simulink model "Simulation_Model1"  (R2020a)
settings: Solver=FixedStepAuto  StartTime=0.0  StopTime=6  FixedStep=.01  RelTol=1e-3
values from neighbouring files (symbols this model uses):
  Mot = F15_Motor    [Simulation_Init.m]
  Veh = Vehicle    [Simulation_Init.m]
libraries: simulink x4, Drag_ul x1, Gravity_ul x1, CgCp_ul x1, NormalForce_ul x1, ThrustCurve_ul x1, Environment_cl x1, Scope_ul x1
settings Model: Creator=bunce  LastModifiedBy=bunce
settings DataIOCC: ReturnWorkspaceOutputs=off
settings SFSimCC: CustomCodeUndefinedFunction=UseInterfaceOnly

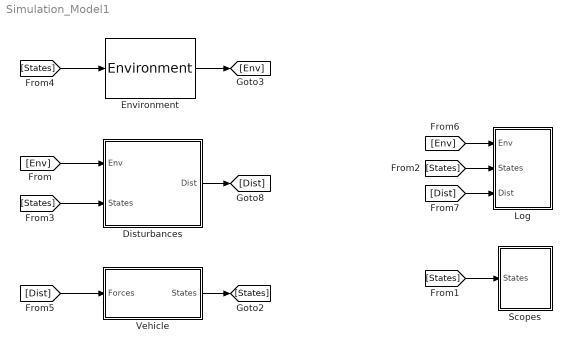
== system Simulation_Model1 ==
  Disturbances : Subsystem
      mask Display:
      | patch([0 1 1 0], [0 0 1 1],[1 .85 1])
      | 
      | port_label('input',1,'Env','texmode','on')
      | 
      | port_label('input',2,'States','texmode','on')
      | 
      | port_label('output',1,'Dist','texmode','on')
  Environment : Environment_cl/Environment  SystemSampleTime=-1  Latency=0  AutoFrameSizeCalculation=off
  Log : Subsystem
      mask Display:
      | patch([0 1 1 0], [0 0 1 1],[1 .85 1])
      | 
      | port_label('input',1,'Env','texmode','on')
      | 
      | port_label('input',2,'States','texmode','on')
      | 
      | port_label('input',3,'Dist','texmode','on')
  Scopes : Subsystem
      mask Display:
      | patch([0 1 1 0], [0 0 1 1],[1 .85 1])
      | 
      | port_label('input',1,'States','texmode','on')
  Vehicle : Subsystem
  wires:
  [Dist] -> Vehicle/1("Forces ")
  Vehicle/1("States ") -> [States]
  [Env] -> Disturbances/1("Env ")
  [States] -> Disturbances/2("States ")
  Disturbances/1(Dist) -> [Dist]
  Environment/1 -> [Env]
  [States] -> Environment/1
  [Dist] -> Log/3(Dist)
  [States] -> Log/2(States)
  [Env] -> Log/1(Env)
  [States] -> Scopes/1(States)

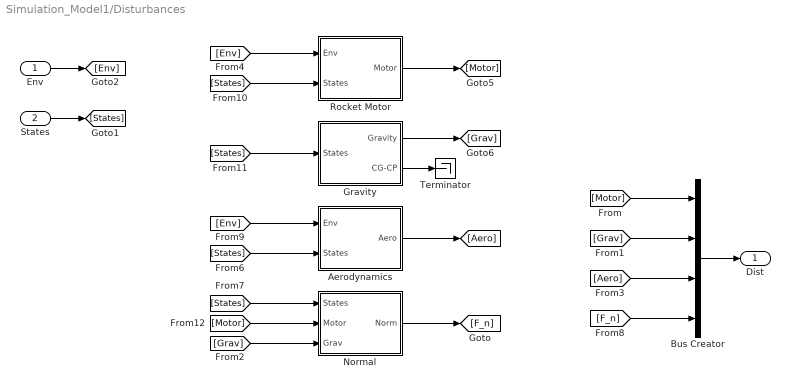
== system Simulation_Model1/Disturbances ==
  "Env " : Inport
  "States " : Inport  Port=2
  Aerodynamics : Subsystem
      mask Display:
      | patch([0 1 1 0], [0 0 1 1],[1 .85 1])
      | 
      | port_label('input',1,'Env','texmode','on')
      | 
      | port_label('input',2,'States', 'texmode','on')
      | 
      | port_label('output',1,'Aero','texmode','on')
  Bus Creator : BusCreator  Inputs=4
  Gravity : Subsystem
      mask Display:
      | patch([0 1 1 0], [0 0 1 1],[1 .85 1])
      | 
      | port_label('input',1,'States','texmode','on')
      | 
      | 
      | port_label('output',1,'Grav','texmode','on')
      | 
      | port_label('output',2,'CG-CP','texmode','on')
  Normal : Subsystem
      mask Display:
      | patch([0 1 1 0], [0 0 1 1],[1 .85 1])
      | 
      | port_label('input',1,'States','texmode','on')
      | 
      | port_label('input',2,'Motor', 'texmode','on')
      | 
      | port_label('input',3,'Grav', 'texmode','on')
      | 
      | port_label('output',1,'F_n','texmode','on')
  Rocket Motor : Subsystem
      mask Display:
      | patch([0 1 1 0], [0 0 1 1],[1 .85 1])
      | 
      | port_label('input',1,'Env','texmode','on')
      | 
      | port_label('input',2,'States', 'texmode','on')
      | 
      | port_label('output',1,'Motor','texmode','on')
  Terminator : Terminator
  Dist : Outport  VectorParamsAs1DForOutWhenUnconnected=off
  wires:
  "States "/1 -> [States]
  [Motor] -> Bus Creator/1
  [Grav] -> Bus Creator/2
  [Aero] -> Bus Creator/3
  [F_n] -> Bus Creator/4
  Bus Creator/1 -> Dist/1
  "Env "/1 -> [Env]
  [States] -> Aerodynamics/2(States)
  [Env] -> Aerodynamics/1(Env)
  Aerodynamics/1(Aero) -> [Aero]
  [Env] -> Rocket Motor/1(Env)
  Rocket Motor/1(Motor) -> [Motor]
  [States] -> Rocket Motor/2(States)
  Gravity/1(Gravity) -> [Grav]
  [States] -> Gravity/1(States)
  [States] -> Normal/1(States)
  [Motor] -> Normal/2(Motor)
  [Grav] -> Normal/3(Grav)
  Normal/1(Norm) -> [F_n]
  Gravity/2(CG-CP) -> Terminator/1

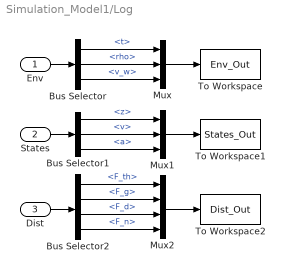
== system Simulation_Model1/Log ==
  Env : Inport
  States : Inport  Port=2
  Dist : Inport  Port=3
  Bus Selector : BusSelector  OutputSignals=t,rho,v_w
  Bus Selector1 : BusSelector  OutputSignals=z,v,a
  Bus Selector2 : BusSelector  OutputSignals=Motor.F_th,Gravity.F_g,Aero.F_d,Norm.F_n
  Mux : Mux  Inputs=3
  Mux1 : Mux  Inputs=3
  Mux2 : Mux
  To Workspace : ToWorkspace  VariableName=Env_Out  SaveFormat=Structure With Time  SampleTime=-1
  To Workspace1 : ToWorkspace  VariableName=States_Out  SaveFormat=Structure With Time  SampleTime=-1
  To Workspace2 : ToWorkspace  VariableName=Dist_Out  SaveFormat=Structure With Time  SampleTime=-1
  wires:
  Env/1 -> Bus Selector/1
  States/1 -> Bus Selector1/1
  Dist/1 -> Bus Selector2/1
  Bus Selector1/3 -> Mux1/3  "<a>"
  Bus Selector1/2 -> Mux1/2  "<v>"
  Bus Selector2/2 -> Mux2/2  "<F_g>"
  Bus Selector2/3 -> Mux2/3  "<F_d>"
  Bus Selector2/4 -> Mux2/4  "<F_n>"
  Bus Selector2/1 -> Mux2/1  "<F_th>"
  Bus Selector1/1 -> Mux1/1  "<z>"
  Bus Selector/1 -> Mux/1  "<t>"
  Bus Selector/2 -> Mux/2  "<rho>"
  Bus Selector/3 -> Mux/3  "<v_w>"
  Mux/1 -> To Workspace/1
  Mux1/1 -> To Workspace1/1
  Mux2/1 -> To Workspace2/1

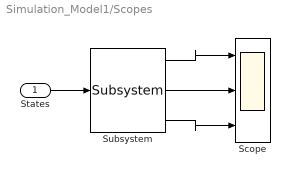
== system Simulation_Model1/Scopes ==
  States : Inport
  Scope : Scope  NumInputPorts=3
  Subsystem : Scope_ul/Subsystem  SystemSampleTime=-1  Latency=0  AutoFrameSizeCalculation=off
      mask Display:
      | patch([0 1 1 0], [0 0 1 1],[.8 1 1])
      | 
      | port_label('input',1,'States','texmode','on')
      | 
      | port_label('output',1,'z [m]','texmode','on')
      | 
      | port_label('output',2,'v [m/s]','texmode','on')
      | 
      | port_label('output',3,'a [m/s^2]','texmode','on')
  wires:
  States/1 -> Subsystem/1
  Subsystem/1 -> Scope/1
  Subsystem/2 -> Scope/2
  Subsystem/3 -> Scope/3

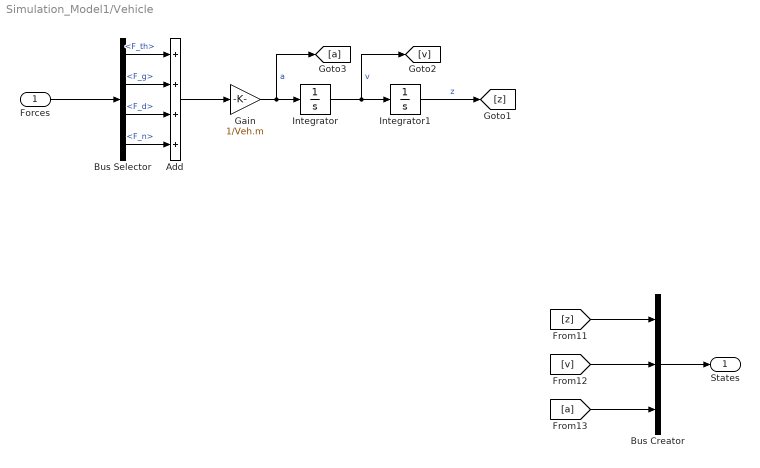
== system Simulation_Model1/Vehicle ==
  "Forces " : Inport
  Add : Sum  Inputs=++++
  Bus Creator : BusCreator  Inputs=3
  Bus Selector : BusSelector  OutputSignals=Motor.F_th,Gravity.F_g,Aero.F_d,Norm.F_n
  Gain : Gain  Gain=1/Veh.m
  Integrator : Integrator
  Integrator1 : Integrator  LimitOutput=on  LowerSaturationLimit=0
  "States " : Outport  VectorParamsAs1DForOutWhenUnconnected=off
  wires:
  [a] -> Bus Creator/3
  [v] -> Bus Creator/2
  [z] -> Bus Creator/1
  Bus Creator/1 -> "States "/1
  Bus Selector/4 -> Add/4  "<F_n>"
  Gain/1 -> [a], Integrator/1  "a"
  Add/1 -> Gain/1
  Bus Selector/2 -> Add/2  "<F_g>"
  Bus Selector/3 -> Add/3  "<F_d>"
  Bus Selector/1 -> Add/1  "<F_th>"
  Integrator1/1 -> [z]  "z"
  Integrator/1 -> Integrator1/1, [v]  "v"
  "Forces "/1 -> Bus Selector/1

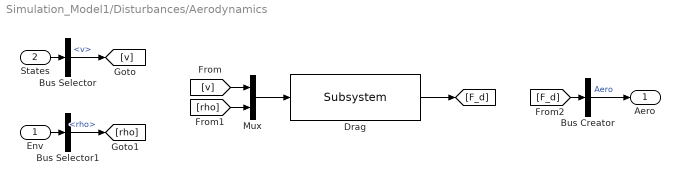
== system Simulation_Model1/Disturbances/Aerodynamics ==
  Env : Inport
  States : Inport  Port=2
  Bus Creator : BusCreator  Inputs=1
  Bus Selector : BusSelector  OutputSignals=v
  Bus Selector1 : BusSelector  OutputSignals=rho
  Drag : Drag_ul/Subsystem  SystemSampleTime=-1  Latency=0  AutoFrameSizeCalculation=off
      mask Display:
      | patch([0 1 1 0], [0 0 1 1],[.8 1 1])
      | 
      | port_label('input',1,'v [m/s], \rho [kg/m^2]','texmode','on')
      | 
      | 
      | port_label('output',1,'F_d [N]','texmode','on')
  Mux : Mux  Inputs=2
  Aero : Outport  VectorParamsAs1DForOutWhenUnconnected=off
  wires:
  States/1 -> Bus Selector/1
  Bus Selector/1 -> [v]  "<v>"
  [v] -> Mux/1
  Env/1 -> Bus Selector1/1
  Bus Selector1/1 -> [rho]  "<rho>"
  [rho] -> Mux/2
  Bus Creator/1 -> Aero/1  "Aero"
  [F_d] -> Bus Creator/1
  Mux/1 -> Drag/1
  Drag/1 -> [F_d]

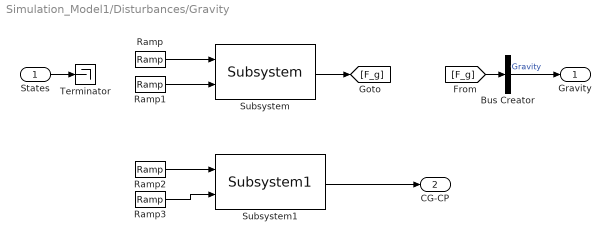
== system Simulation_Model1/Disturbances/Gravity ==
  States : Inport
  Bus Creator : BusCreator  Inputs=1
  Ramp : simulink/Sources/Ramp  slope=-Mot.m_f/Mot.t_b  start=0  InitialOutput=Veh.m+Mot.m
  Ramp1 : simulink/Sources/Ramp  slope=Mot.m_f/Mot.t_b  start=Mot.t_b  InitialOutput=0
  Ramp2 : simulink/Sources/Ramp  slope=-(Veh.L_CG)/Mot.t_b  start=0  InitialOutput=Veh.CG_1
  Ramp3 : simulink/Sources/Ramp  slope=(Veh.L_CG)/Mot.t_b  start=Mot.t_b  InitialOutput=0
  Subsystem : Gravity_ul/Subsystem  SystemSampleTime=-1  Latency=0  AutoFrameSizeCalculation=off
      mask Display:
      | patch([0 1 1 0], [0 0 1 1],[.8 1 1])
      | 
      | port_label('input',1,'Mass_M [Kg]','texmode','on')
      | 
      | port_label('input',2,'Mass_M [Kg]','texmode','on')
      | 
      | port_label('output',1,'F_{g} [N]','texmode','on')
  Subsystem1 : CgCp_ul/Subsystem1  SystemSampleTime=-1  Latency=0  AutoFrameSizeCalculation=off
      mask Display:
      | patch([0 1 1 0], [0 0 1 1],[.8 1 1])
      | 
      | port_label('input',1,'Mass_M [Kg]','texmode','on')
      | 
      | port_label('input',2,'Mass_M [Kg]','texmode','on')
      | 
      | port_label('output',1,'C_{g}-C_p [N]','texmode','on')
  Terminator : Terminator
  Gravity : Outport  VectorParamsAs1DForOutWhenUnconnected=off
  CG-CP : Outport  Port=2  VectorParamsAs1DForOutWhenUnconnected=off
  wires:
  States/1 -> Terminator/1
  [F_g] -> Bus Creator/1
  Bus Creator/1 -> Gravity/1  "Gravity"
  Subsystem/1 -> [F_g]
  Ramp/1 -> Subsystem/1
  Ramp1/1 -> Subsystem/2
  Ramp2/1 -> Subsystem1/1
  Ramp3/1 -> Subsystem1/2
  Subsystem1/1 -> CG-CP/1

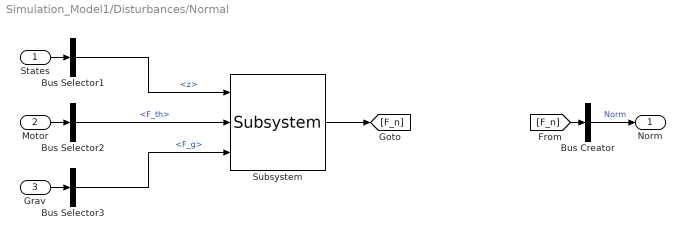
== system Simulation_Model1/Disturbances/Normal ==
  States : Inport
  Motor : Inport  Port=2
  Grav : Inport  Port=3
  Bus Creator : BusCreator  Inputs=1
  Bus Selector1 : BusSelector  OutputSignals=z
  Bus Selector2 : BusSelector  OutputSignals=F_th
  Bus Selector3 : BusSelector  OutputSignals=F_g
  Subsystem : NormalForce_ul/Subsystem  SystemSampleTime=-1  Latency=0  AutoFrameSizeCalculation=off
      mask Display:
      | patch([0 1 1 0], [0 0 1 1],[.8 1 1])
      | 
      | port_label('input',1,'z [m]', 'texmode','on')
      | 
      | port_label('input',2,'F_{th} [N]','texmode','on')
      | 
      | port_label('input',3,'F_g [N]','texmode','on')
      | 
      | 
      | port_label('output',1,'F_n [N]','texmode','on')
  Norm : Outport  VectorParamsAs1DForOutWhenUnconnected=off
  wires:
  States/1 -> Bus Selector1/1
  Motor/1 -> Bus Selector2/1
  Grav/1 -> Bus Selector3/1
  [F_n] -> Bus Creator/1
  Bus Creator/1 -> Norm/1  "Norm"
  Bus Selector1/1 -> Subsystem/1  "<z>"
  Bus Selector2/1 -> Subsystem/2  "<F_th>"
  Bus Selector3/1 -> Subsystem/3  "<F_g>"
  Subsystem/1 -> [F_n]

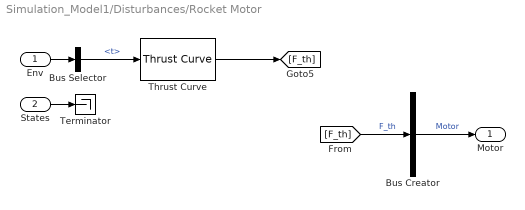
== system Simulation_Model1/Disturbances/Rocket Motor ==
  Env : Inport
  States : Inport  Port=2
  Bus Creator : BusCreator  Inputs=1
  Bus Selector : BusSelector  OutputSignals=t
  Terminator : Terminator
  Thrust Curve : ThrustCurve_ul/Thrust Curve  SystemSampleTime=-1  Latency=0  AutoFrameSizeCalculation=off
      mask Display:
      | patch([0 1 1 0], [0 0 1 1],[.8 1 1])
      | 
      | port_label('input',1,'t [s]','texmode','on')
      | 
      | port_label('output',1,'F_{th} [N]','texmode','on')
  Motor : Outport  VectorParamsAs1DForOutWhenUnconnected=off
  wires:
  Env/1 -> Bus Selector/1
  States/1 -> Terminator/1
  Bus Creator/1 -> Motor/1  "Motor"
  [F_th] -> Bus Creator/1  "F_th"
  Bus Selector/1 -> Thrust Curve/1  "<t>"
  Thrust Curve/1 -> [F_th]
